simulink model "dec_dly_comp"  (R2023b)
settings: Solver=VariableStepDiscrete  StartTime=0.0  StopTime=DDC_LINEUP_param.endTime  RelTol=1e-3  EnableMultiTasking=on
PreLoadFcn:
  | % Run the setup script when the model is opened
  | setup_dec_dly_comp;
InitFcn:
  | % Run the setup script again just before the
  | % model is run, so that any updates made
  | % after opening are applied.
  | 
  | setup_dec_dly_comp;
StopFcn:
  | dec_dly_comp_output_analysis;
undefined symbols (not defined in the file or in its folder): AdvDSPBChannelOutDisplay, AdvDSPBDMemDisplay, DDC_LINEUP_param, dpoly, dspba_ChannelInVis, dspba_ChannelOutVis, dspba_internal_get_channel_ports, evalAionMaskParam, latency, primtype, UseDontCare, value
libraries: DSPBAPrim x52, DSPBAModelBus x14, DSPBABase x10, simulink x9, DSPBAFilters x2
(part 1 of 2)
Description:
  | DSP Builder Advanced Template for Template Design implementing ModelIP designs
settings Model: Creator=mjervis  LastModifiedBy=5g
settings SolverCC: AlgebraicLoopSolver=TrustRegion
settings DataIOCC: LimitDataPoints=on  SaveFormat=Array  SignalLoggingSaveFormat=ModelDataLogs  ReturnWorkspaceOutputs=off
settings OptimizationCC: ExpressionDepthLimit=2147483647  LifeSpan=inf
settings DebuggingCC: UnderspecifiedInitializationDetection=Classic  MergeDetectMultiDrivingBlocksExec=none  SolverPrmCheckMsg=warning  InheritedTsInSrcMsg=none  IntegerOverflowMsg=none  FcnCallInpInsideContextMsg=warning  UnconnectedInputMsg=warning  UnconnectedOutputMsg=warning  UnconnectedLineMsg=warning  StateNameClashWarn=warning  SFUnexpectedBacktrackingDiag=warning  SFNoUnconditionalDefaultTransitionDiag=warning  SFExecutionAtInitializationDiag=none  IntegerSaturationMsg=none  ArithmeticOperatorsInVariantConditions=warning
settings HardwareCC: ProdBitPerPointer=32  ProdBitPerSizeT=32  ProdBitPerPtrDiffT=32  ProdLargestAtomicFloat=None  ProdIntDivRoundTo=Undefined  ProdEndianess=Unspecified  ProdWordSize=32  ProdHWDeviceType=32-bit Generic
settings ModelReferenceCC: EnableRefExpFcnMdlSchedulingChecks=on  PropagateSignalLabelsOutOfModel=off
settings SFSimCC: SimUseLocalCustomCode=off  CustomCodeUndefinedFunction=UseInterfaceOnly
settings RTWCC: RTWUseLocalCustomCode=off  DLArmComputeVersion=19.05
settings CodeAppCC: StateflowObjectComments=on
settings GRTTargetCC: TargetLangStandard=C89/C90 (ANSI)  CombineOutputUpdateFcns=off  GRTInterface=on
settings ConfigComp: CovMetricSettings=dw  CovSaveCumulativeToWorkspaceVar=on  CovSaveSingleToWorkspaceVar=on  CovExternalEMLEnable=off

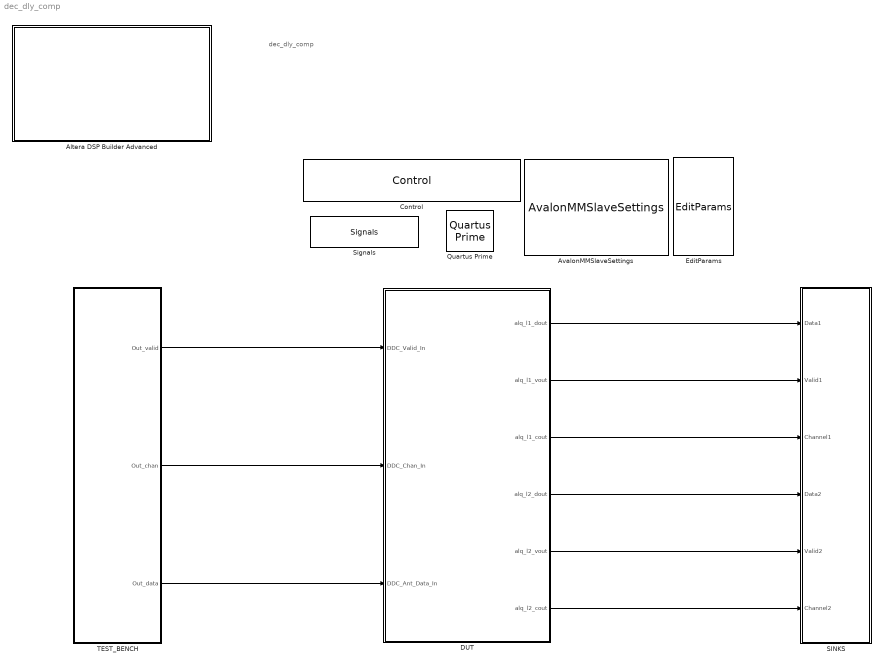
== system dec_dly_comp ==
  note: dec_dly_comp
  Altera DSP Builder Advanced : Subsystem  mask(DSP Builder Advanced Blockset Ignored Block){}
      settings: OpenFcn=web('http://www.altera.com', '-new');
      mask Display: image(imread('intellogo.tif'));
  AvalonMMSlaveSettings : DSPBABase/AvalonMMSlaveSettings
  Control : DSPBABase/Control  generate=on  language=VHDL  destination=./rtl  destination_gui=./rtl  make_full_path=off  path_is_relative=on  autotestbench=on  signaldepth=2  coveragetestbench=off  logs=off  spacewidth=2  spacenum=1  addrwidth=14  datawidth=32  dataendian=Big Endian  hierarchicalnames=off  ramThresholdBits=-1  distRamThresholdBits=-1  mlabThresholdBits=-1  hardMultiplierThresholdLuts=-1  version=20090407  errorOnChanMismatch=1  errorOnGPIOMismatch=0  importModelsimResults=0  cycleAccurate=off  reinterpretCastMult=off  paramFile=dec_dly_comp_params.xml
  DUT : Subsystem
  EditParams : DSPBABase/EditParams  version=20090407
  Quartus Prime : DSPBABase/Quartus Prime  version=20090407
  SINKS : Subsystem
  Signals : DSPBABase/Signals  clk=clk  freq=240  margin=0  rst=areset  rstactive=High  bus=bus  enbusclock=off  busfreq=491.52  bussync=off  version=20090407
  TEST_BENCH : Subsystem
  wires:
  DUT/1(alq_l1_dout) -> SINKS/1(Data1)
  DUT/2(alq_l1_vout) -> SINKS/2(Valid1)
  DUT/3("alq_l1_cout ") -> SINKS/3(Channel1)
  DUT/4(alq_l2_dout) -> SINKS/4(Data2)
  DUT/5(alq_l2_vout) -> SINKS/5(Valid2)
  DUT/6(alq_l2_cout) -> SINKS/6(Channel2)
  TEST_BENCH/1(Out_valid) -> DUT/1(DDC_Valid_In)
  TEST_BENCH/2(Out_chan) -> DUT/2(DDC_Chan_In)
  TEST_BENCH/3(Out_data) -> DUT/3(DDC_Ant_Data_In)

== system dec_dly_comp/Altera DSP Builder Advanced ==

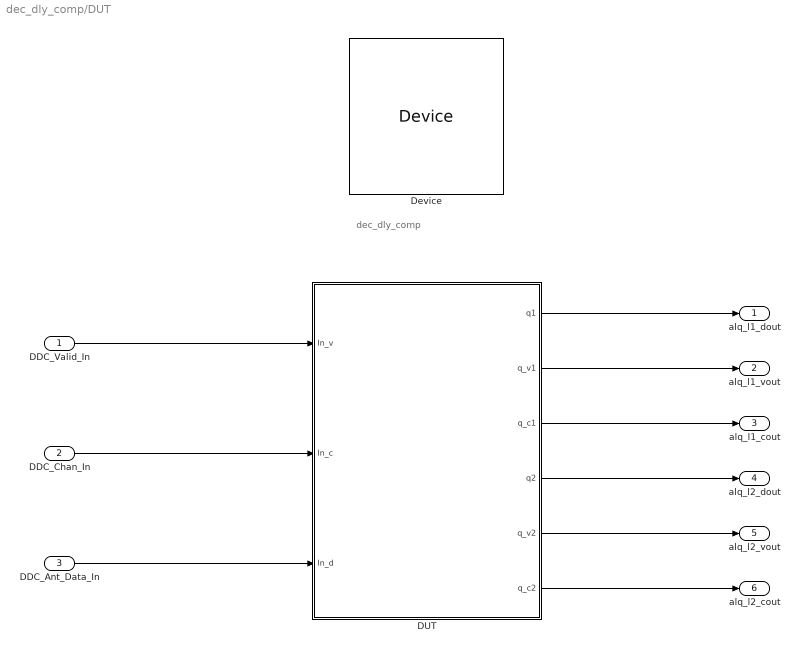
== system dec_dly_comp/DUT ==
  note: dec_dly_comp
  DDC_Valid_In : Inport
  DDC_Chan_In : Inport  Port=2
  DDC_Ant_Data_In : Inport  Port=3
  DUT : Subsystem
  Device : DSPBABase/Device  family=Arria 10  deviceMember=Stratix V GX  stratix4device=Stratix IV GX  hardcopy4device=HardCopy IV E  stratix5device=Stratix V GX  device=10AS066N2F40I1SGES  speed=1  stratixSpeed=-5  stratix2Speed=-3  stratix3Speed=-3  stratix4gxSpeed=-2  stratix4gtSpeed=-1  cyclone2Speed=-6  cyclone3Speed=-7  arria2Speed=-4  cyclone4eSpeed=-8  stratix5Speed=-3  arria5Speed=-4  arriaSpeed=-6  cyclone3lsSpeed=-7  cyclone5Speed=-6  arria2gzSpeed=-3  nightFurySpeed=-2  ecp2Speed=-7  hardcopycompat=off  version=20140217  max10flashmode=off  max10nomeminit=off
  alq_l1_dout : Outport
  alq_l1_vout : Outport  Port=2
  "alq_l1_cout " : Outport  Port=3
  alq_l2_dout : Outport  Port=4
  alq_l2_vout : Outport  Port=5
  alq_l2_cout : Outport  Port=6
  wires:
  DDC_Valid_In/1 -> DUT/1(In_v)
  DDC_Chan_In/1 -> DUT/2(In_c)
  DDC_Ant_Data_In/1 -> DUT/3(In_d)
  DUT/2(q_v1) -> alq_l1_vout/1
  DUT/1(q1) -> alq_l1_dout/1
  DUT/3(q_c1) -> "alq_l1_cout "/1
  DUT/5(q_v2) -> alq_l2_vout/1
  DUT/6(q_c2) -> alq_l2_cout/1
  DUT/4(q2) -> alq_l2_dout/1

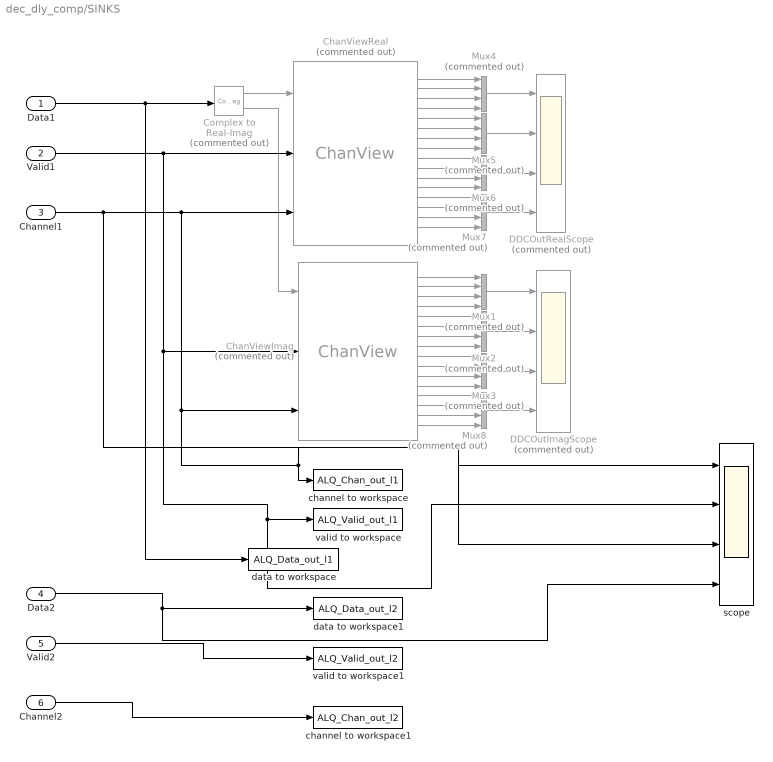
== system dec_dly_comp/SINKS ==
  Data1 : Inport
  Valid1 : Inport  Port=2
  Channel1 : Inport  Port=3
  Data2 : Inport  Port=4
  Valid2 : Inport  Port=5
  Channel2 : Inport  Port=6
  ChanViewImag : DSPBABase/ChanView  Commented=on  nchans=16  chan_vector=[0:15]  outsvalid=off  latency=1  version=20090407
  ChanViewReal : DSPBABase/ChanView  Commented=on  nchans=16  chan_vector=[0:15]  outsvalid=off  latency=1  version=20090407
  Complex to Real-Imag : ComplexToRealImag  Commented=on
  DDCOutImagScope : Scope  Commented=on  NumInputPorts=4
  DDCOutRealScope : Scope  Commented=on  NumInputPorts=4
  Mux{1..8} (8 alike) : Mux  Commented=on
  channel to workspace : ToWorkspace  VariableName=ALQ_Chan_out_l1  SaveFormat=Timeseries  SampleTime=-1
  channel to workspace1 : ToWorkspace  VariableName=ALQ_Chan_out_l2  SaveFormat=Timeseries  SampleTime=-1
  data to workspace : ToWorkspace  VariableName=ALQ_Data_out_l1  SaveFormat=Timeseries  SampleTime=-1
  data to workspace1 : ToWorkspace  VariableName=ALQ_Data_out_l2  SaveFormat=Timeseries  SampleTime=-1
  scope : Scope  NumInputPorts=4
  valid to workspace : ToWorkspace  VariableName=ALQ_Valid_out_l1  SaveFormat=Timeseries  SampleTime=-1
  valid to workspace1 : ToWorkspace  VariableName=ALQ_Valid_out_l2  SaveFormat=Timeseries  SampleTime=-1
  wires:
  Mux7/1 -> DDCOutRealScope/4
  ChanViewReal/14 -> Mux7/2
  ChanViewReal/15 -> Mux7/3
  ChanViewReal/16 -> Mux7/4
  ChanViewReal/13 -> Mux7/1
  Mux6/1 -> DDCOutRealScope/3
  ChanViewReal/11 -> Mux6/3
  ChanViewReal/12 -> Mux6/4
  ChanViewReal/9 -> Mux6/1
  ChanViewReal/10 -> Mux6/2
  Mux5/1 -> DDCOutRealScope/2
  ChanViewReal/6 -> Mux5/2
  ChanViewReal/7 -> Mux5/3
  ChanViewReal/5 -> Mux5/1
  ChanViewReal/8 -> Mux5/4
  Mux4/1 -> DDCOutRealScope/1
  ChanViewReal/3 -> Mux4/3
  ChanViewReal/4 -> Mux4/4
  ChanViewReal/2 -> Mux4/2
  ChanViewReal/1 -> Mux4/1
  Complex to Real-Imag/2 -> ChanViewImag/1
  Complex to Real-Imag/1 -> ChanViewReal/1
  Data1/1 -> data to workspace/1, Complex to Real-Imag/1
  Channel1/1 -> scope/3, scope/1, channel to workspace/1, ChanViewImag/3, ChanViewReal/3
  Valid1/1 -> ChanViewReal/2, scope/2, valid to workspace/1, ChanViewImag/2
  Mux8/1 -> DDCOutImagScope/4
  ChanViewImag/14 -> Mux8/2
  ChanViewImag/15 -> Mux8/3
  ChanViewImag/16 -> Mux8/4
  ChanViewImag/13 -> Mux8/1
  Mux3/1 -> DDCOutImagScope/3
  ChanViewImag/11 -> Mux3/3
  ChanViewImag/12 -> Mux3/4
  ChanViewImag/9 -> Mux3/1
  ChanViewImag/10 -> Mux3/2
  Mux2/1 -> DDCOutImagScope/2
  ChanViewImag/6 -> Mux2/2
  ChanViewImag/7 -> Mux2/3
  ChanViewImag/5 -> Mux2/1
  ChanViewImag/8 -> Mux2/4
  Mux1/1 -> DDCOutImagScope/1
  ChanViewImag/3 -> Mux1/3
  ChanViewImag/4 -> Mux1/4
  ChanViewImag/2 -> Mux1/2
  ChanViewImag/1 -> Mux1/1
  Data2/1 -> scope/4, data to workspace1/1
  Valid2/1 -> valid to workspace1/1
  Channel2/1 -> channel to workspace1/1

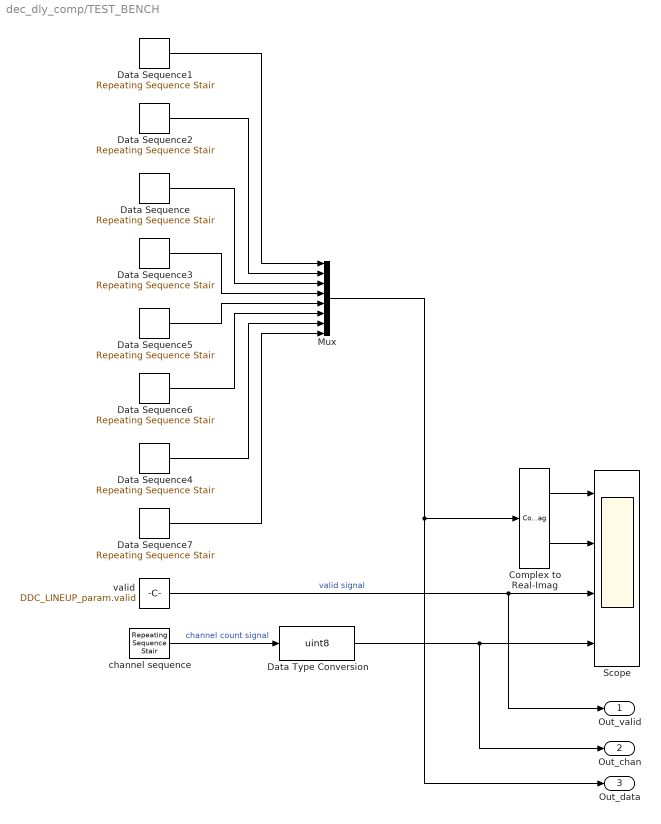
== system dec_dly_comp/TEST_BENCH ==
  Complex to Real-Imag : ComplexToRealImag
  Data Sequence : simulink/Sources/Repeating Sequence Stair  OutValues=DDC_LINEUP_param.DDC_Ant_Data_in_3  tsamp=DDC_LINEUP_param.SampleTime  OutMin=[]  OutMax=[]  OutDataTypeStr=fixdt(1,16,14)  OutputDataTypeScalingMode=Specify via dialog  OutDataType=fixdt(1,16,14)  ConRadixGroup=Best Precision: Vector-wise  OutScaling=[]
  Data Sequence1 : simulink/Sources/Repeating Sequence Stair  OutValues=DDC_LINEUP_param.DDC_Ant_Data_in_1  tsamp=DDC_LINEUP_param.SampleTime  OutMin=[]  OutMax=[]  OutDataTypeStr=fixdt(1,16,14)  OutputDataTypeScalingMode=Specify via dialog  OutDataType=fixdt(1,16,14)  ConRadixGroup=Best Precision: Vector-wise  OutScaling=[]
  Data Sequence2 : simulink/Sources/Repeating Sequence Stair  OutValues=DDC_LINEUP_param.DDC_Ant_Data_in_2  tsamp=DDC_LINEUP_param.SampleTime  OutMin=[]  OutMax=[]  OutDataTypeStr=fixdt(1,16,14)  OutputDataTypeScalingMode=Specify via dialog  OutDataType=fixdt(1,16,14)  ConRadixGroup=Best Precision: Vector-wise  OutScaling=[]
  Data Sequence3 : simulink/Sources/Repeating Sequence Stair  OutValues=DDC_LINEUP_param.DDC_Ant_Data_in_4  tsamp=DDC_LINEUP_param.SampleTime  OutMin=[]  OutMax=[]  OutDataTypeStr=fixdt(1,16,14)  OutputDataTypeScalingMode=Specify via dialog  OutDataType=fixdt(1,16,14)  ConRadixGroup=Best Precision: Vector-wise  OutScaling=[]
  Data Sequence4 : simulink/Sources/Repeating Sequence Stair  OutValues=DDC_LINEUP_param.DDC_Ant_Data_in_7  tsamp=DDC_LINEUP_param.SampleTime  OutMin=[]  OutMax=[]  OutDataTypeStr=fixdt(1,16,14)  OutputDataTypeScalingMode=Specify via dialog  OutDataType=fixdt(1,16,14)  ConRadixGroup=Best Precision: Vector-wise  OutScaling=[]
  Data Sequence5 : simulink/Sources/Repeating Sequence Stair  OutValues=DDC_LINEUP_param.DDC_Ant_Data_in_5  tsamp=DDC_LINEUP_param.SampleTime  OutMin=[]  OutMax=[]  OutDataTypeStr=fixdt(1,16,14)  OutputDataTypeScalingMode=Specify via dialog  OutDataType=fixdt(1,16,14)  ConRadixGroup=Best Precision: Vector-wise  OutScaling=[]
  Data Sequence6 : simulink/Sources/Repeating Sequence Stair  OutValues=DDC_LINEUP_param.DDC_Ant_Data_in_6  tsamp=DDC_LINEUP_param.SampleTime  OutMin=[]  OutMax=[]  OutDataTypeStr=fixdt(1,16,14)  OutputDataTypeScalingMode=Specify via dialog  OutDataType=fixdt(1,16,14)  ConRadixGroup=Best Precision: Vector-wise  OutScaling=[]
  Data Sequence7 : simulink/Sources/Repeating Sequence Stair  OutValues=DDC_LINEUP_param.DDC_Ant_Data_in_8  tsamp=DDC_LINEUP_param.SampleTime  OutMin=[]  OutMax=[]  OutDataTypeStr=fixdt(1,16,14)  OutputDataTypeScalingMode=Specify via dialog  OutDataType=fixdt(1,16,14)  ConRadixGroup=Best Precision: Vector-wise  OutScaling=[]
  Data Type Conversion : DataTypeConversion  OutDataTypeStr=uint8  SaturateOnIntegerOverflow=off  RndMeth=Floor
  Mux : Mux  Inputs=8
  Scope : Scope  NumInputPorts=4
  channel sequence : simulink/Sources/Repeating Sequence Stair  OutValues=DDC_LINEUP_param.channel  tsamp=DDC_LINEUP_param.SampleTime  OutMin=[]  OutMax=[]  OutDataTypeStr=uint8  OutputDataTypeScalingMode=uint8  OutDataType=fixdt(1,16)  ConRadixGroup=Best Precision: Vector-wise  OutScaling=[]
  valid : Constant  Value=DDC_LINEUP_param.valid  OutDataTypeStr=boolean  SampleTime=DDC_LINEUP_param.SampleTime
  Out_valid : Outport
  Out_chan : Outport  Port=2
  Out_data : Outport  Port=3
  wires:
  Complex to Real-Imag/1 -> Scope/1
  valid/1 -> Scope/3, Out_valid/1  "valid signal"
  channel sequence/1 -> Data Type Conversion/1  "channel count signal"
  Data Type Conversion/1 -> Scope/4, Out_chan/1
  Complex to Real-Imag/2 -> Scope/2
  Mux/1 -> Complex to Real-Imag/1, Out_data/1
  Data Sequence5/1 -> Mux/5
  Data Sequence3/1 -> Mux/4
  Data Sequence6/1 -> Mux/6
  Data Sequence/1 -> Mux/3
  Data Sequence4/1 -> Mux/7
  Data Sequence2/1 -> Mux/2
  Data Sequence7/1 -> Mux/8
  Data Sequence1/1 -> Mux/1

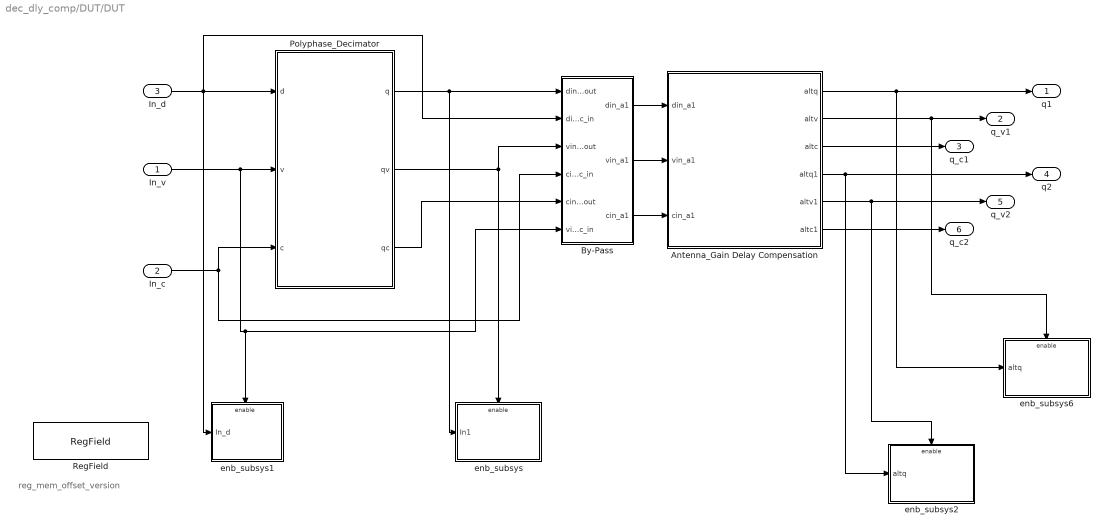
== system dec_dly_comp/DUT/DUT ==
  note: reg_mem_offset_version
  In_v : Inport
  In_c : Inport  Port=2
  In_d : Inport  Port=3
  Antenna_Gain Delay Compensation : Subsystem
  By-Pass : Subsystem
  Polyphase_Decimator : Subsystem
  RegField : DSPBAModelBus/RegField  reg_name=DDC_LINEUP_param.reg_version.mem_offset  reg_rwmode=Read/Write  reg_msb=31  reg_lsb=0  reg_mode=Specify via dialog  reg_type=ufix(32)  reg_scale=2^0  reg_init=DDC_LINEUP_param.reg_version.Version_reg_val  reg_desc=Version_Output  reg_modal=off  reg_desc0=0  reg_desc1=0  reg_desc2=0  reg_desc3=0  reg_desc4=0  reg_desc5=0  reg_desc6=0  reg_desc7=0  reg_addr=13  SampleTime=-1  version=20090407
  enb_subsys : Subsystem
  enb_subsys1 : Subsystem
  enb_subsys2 : Subsystem
  enb_subsys6 : Subsystem
  q1 : Outport
  q_v1 : Outport  Port=2
  q_c1 : Outport  Port=3
  q2 : Outport  Port=4
  q_v2 : Outport  Port=5
  q_c2 : Outport  Port=6
  wires:
  Polyphase_Decimator/2(qv) -> enb_subsys/Enable, By-Pass/3(vin_dec_out)
  Polyphase_Decimator/1(q) -> enb_subsys/1(In1), By-Pass/1(din_dec_out)
  In_d/1 -> By-Pass/2(din_dec_in), enb_subsys1/1(In_d), Polyphase_Decimator/1(d)
  In_v/1 -> enb_subsys1/Enable, By-Pass/6(vin_dec_in), Polyphase_Decimator/2(v)
  In_c/1 -> By-Pass/4(cin_dec_in), Polyphase_Decimator/3(c)
  Antenna_Gain Delay Compensation/3(altc) -> q_c1/1
  Antenna_Gain Delay Compensation/2(altv) -> enb_subsys6/Enable, q_v1/1
  Antenna_Gain Delay Compensation/1(altq) -> enb_subsys6/1(altq), q1/1
  Polyphase_Decimator/3(qc) -> By-Pass/5(cin_dec_out)
  By-Pass/1(din_a1) -> Antenna_Gain Delay Compensation/1(din_a1)
  By-Pass/2(vin_a1) -> Antenna_Gain Delay Compensation/2(vin_a1)
  By-Pass/3(cin_a1) -> Antenna_Gain Delay Compensation/3(cin_a1)
  Antenna_Gain Delay Compensation/4(altq1) -> enb_subsys2/1(altq), q2/1
  Antenna_Gain Delay Compensation/5(altv1) -> enb_subsys2/Enable, q_v2/1
  Antenna_Gain Delay Compensation/6(altc1) -> q_c2/1

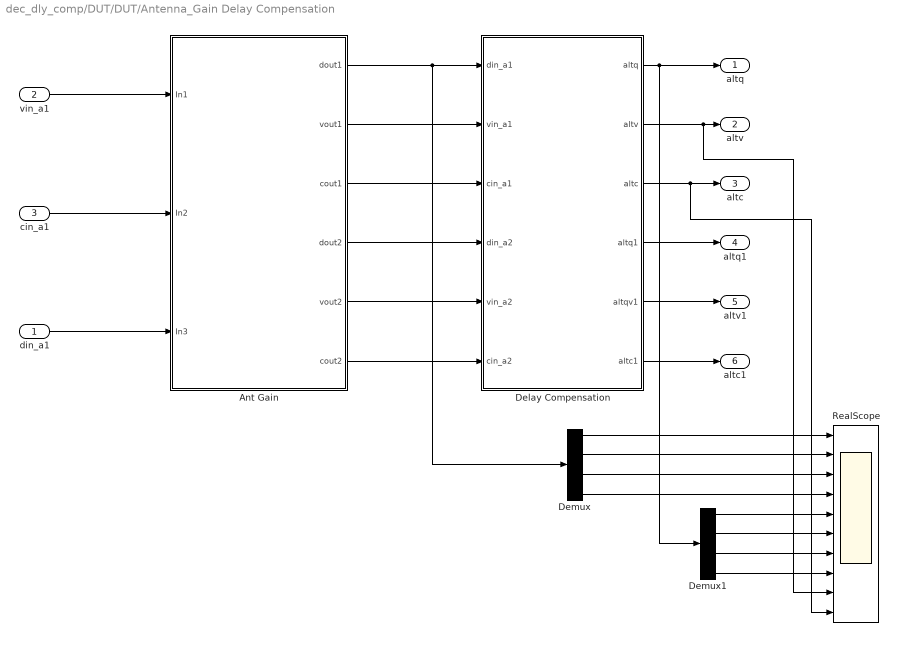
== system dec_dly_comp/DUT/DUT/Antenna_Gain Delay Compensation ==
  din_a1 : Inport
  vin_a1 : Inport  Port=2
  cin_a1 : Inport  Port=3
  Ant Gain : Subsystem
  Delay Compensation : Subsystem
  Demux : Demux
  Demux1 : Demux
  RealScope : Scope  NumInputPorts=10
  altq : Outport
  altv : Outport  Port=2
  altc : Outport  Port=3
  altq1 : Outport  Port=4
  altv1 : Outport  Port=5
  altc1 : Outport  Port=6
  wires:
  vin_a1/1 -> Ant Gain/1(In1)
  cin_a1/1 -> Ant Gain/2(In2)
  din_a1/1 -> Ant Gain/3(In3)
  Ant Gain/3(cout1) -> Delay Compensation/3(cin_a1)
  Ant Gain/2(vout1) -> Delay Compensation/2(vin_a1)
  Ant Gain/4(dout2) -> Delay Compensation/4(din_a2)
  Ant Gain/5(vout2) -> Delay Compensation/5(vin_a2)
  Ant Gain/6(cout2) -> Delay Compensation/6(cin_a2)
  Delay Compensation/4(altq1) -> altq1/1
  Delay Compensation/5(altqv1) -> altv1/1
  Delay Compensation/6(altc1) -> altc1/1
  Ant Gain/1(dout1) -> Demux/1, Delay Compensation/1(din_a1)
  Demux1/2 -> RealScope/6
  Demux/2 -> RealScope/2
  Delay Compensation/2(altv) -> RealScope/9, altv/1
  Demux/1 -> RealScope/1
  Demux1/1 -> RealScope/5
  Demux1/4 -> RealScope/8
  Demux/4 -> RealScope/4
  Demux/3 -> RealScope/3
  Delay Compensation/3(altc) -> RealScope/10, altc/1
  Demux1/3 -> RealScope/7
  Delay Compensation/1(altq) -> altq/1, Demux1/1

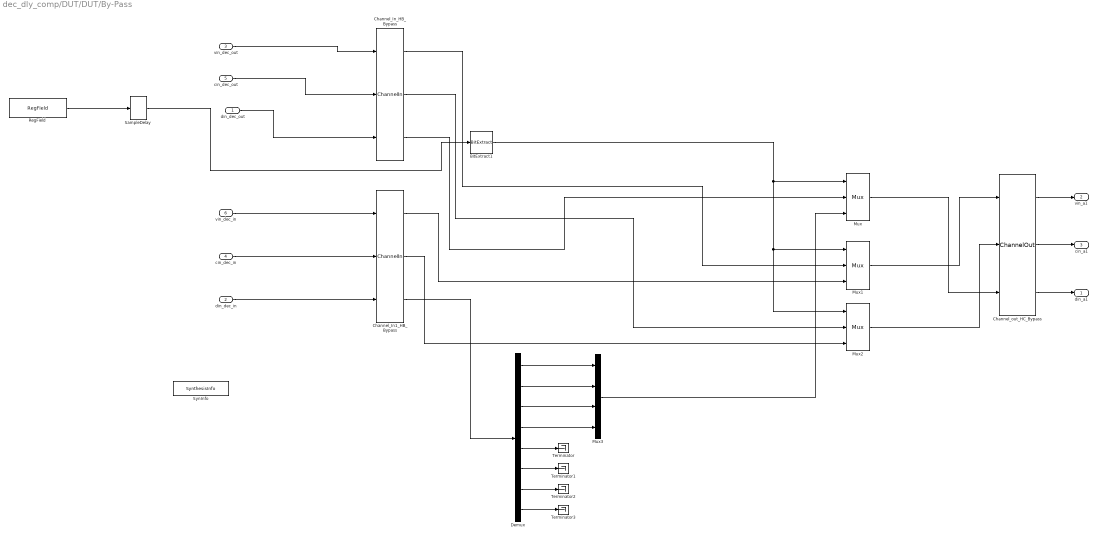
== system dec_dly_comp/DUT/DUT/By-Pass ==
  din_dec_out : Inport
  din_dec_in : Inport  Port=2
  vin_dec_out : Inport  Port=3
  cin_dec_in : Inport  Port=4
  cin_dec_out : Inport  Port=5
  vin_dec_in : Inport  Port=6
  BitExtract1 : DSPBAPrim/BitExtract  primtype=bitextract  nInputs=1  nOutputs=1  omode=boolean  otype=uint(16)  scale=1  rndmethod=Unbiased  factor=1  satmethod=Symmetric  shift_vec=[0 1 2 -1]  value=0  inPortNames=[' '; ' ';]  outPortNames=[' ']  dspbaimage=dspba_prim.svg  text=fprintf('..%d', value);  style=Optimised  visibilities=8+1024  version=20211007
  Channel_In1_HB_Bypass : DSPBAPrim/ChannelIn  primtype=channelin  nInputs=dspba_internal_get_channel_ports(gcb)  nOutputs=dspba_internal_get_channel_ports(gcb)  omode=Inherit via internal rule  otype=sfix(16)  scale=2^-15  rndmethod=Unbiased  factor=1  satmethod=Symmetric  shift_vec=[0 1 2 -1]  value=1  inPortNames=['v'; 'c'; '0'; '1'; '2'; '3'; '4'; '5'; '6'; '7'; '8'; '9'; 'A'; 'B'; 'D'; 'E'; 'F'; 'G'; 'H'; 'I'; 'J'; 'K'; 'L'; 'M'; 'N'; 'O'; 'P'; 'Q'; 'R'; 'S'; 'T'; 'U'; 'W'; 'X'; 'Y'; 'Z']  outPortNames=['v'; 'c'; '0'; '1'; '2'; '3'; '4'; '5'; '6'; '7'; '8'; '9'; 'A'; 'B'; 'D'; 'E'; 'F'; 'G'; 'H'; 'I'; 'J'; 'K'; 'L'; 'M'; 'N'; 'O'; 'P'; 'Q'; 'R'; 'S'; 'T'; 'U'; 'W'; 'X'; 'Y'; 'Z']  dspbaimage=dspba_prim_channel_tall.svg  text=fprintf('In');  style=Optimised  dataSignals=1  foldingEnabled=off  channels=1  sampleRate=200  packetBeginPresent=off  packetBeginEnabled=off  visibilities=dspba_ChannelInVis(gcb)  scheduleOrigin=on  version=20211214
  Channel_In_HB_Bypass : DSPBAPrim/ChannelIn  primtype=channelin  nInputs=dspba_internal_get_channel_ports(gcb)  nOutputs=dspba_internal_get_channel_ports(gcb)  omode=Inherit via internal rule  otype=sfix(16)  scale=2^-15  rndmethod=Unbiased  factor=1  satmethod=Symmetric  shift_vec=[0 1 2 -1]  value=1  inPortNames=['v'; 'c'; '0'; '1'; '2'; '3'; '4'; '5'; '6'; '7'; '8'; '9'; 'A'; 'B'; 'D'; 'E'; 'F'; 'G'; 'H'; 'I'; 'J'; 'K'; 'L'; 'M'; 'N'; 'O'; 'P'; 'Q'; 'R'; 'S'; 'T'; 'U'; 'W'; 'X'; 'Y'; 'Z']  outPortNames=['v'; 'c'; '0'; '1'; '2'; '3'; '4'; '5'; '6'; '7'; '8'; '9'; 'A'; 'B'; 'D'; 'E'; 'F'; 'G'; 'H'; 'I'; 'J'; 'K'; 'L'; 'M'; 'N'; 'O'; 'P'; 'Q'; 'R'; 'S'; 'T'; 'U'; 'W'; 'X'; 'Y'; 'Z']  dspbaimage=dspba_prim_channel_tall.svg  text=fprintf('In');  style=Optimised  dataSignals=1  foldingEnabled=off  channels=1  sampleRate=200  packetBeginPresent=off  packetBeginEnabled=off  visibilities=dspba_ChannelInVis(gcb)  scheduleOrigin=on  version=20211214
  Channel_out_HC_Bypass : DSPBAPrim/ChannelOut  primtype=channelout  nInputs=dspba_internal_get_channel_ports(gcb)  nOutputs=dspba_internal_get_channel_ports(gcb)  omode=Inherit via internal rule  otype=sfix(16)  scale=2^-15  rndmethod=Unbiased  factor=1  satmethod=Symmetric  shift_vec=[0 1 2 -1]  value=1  inPortNames=['v'; 'c'; '0'; '1'; '2'; '3'; '4'; '5'; '6'; '7'; '8'; '9'; 'A'; 'B'; 'D'; 'E'; 'F'; 'G'; 'H'; 'I'; 'J'; 'K'; 'L'; 'M'; 'N'; 'O'; 'P'; 'Q'; 'R'; 'S'; 'T'; 'U'; 'W'; 'X'; 'Y'; 'Z']  outPortNames=['v'; 'c'; '0'; '1'; '2'; '3'; '4'; '5'; '6'; '7'; '8'; '9'; 'A'; 'B'; 'D'; 'E'; 'F'; 'G'; 'H'; 'I'; 'J'; 'K'; 'L'; 'M'; 'N'; 'O'; 'P'; 'Q'; 'R'; 'S'; 'T'; 'U'; 'W'; 'X'; 'Y'; 'Z']  dspbaimage=dspba_prim_channel_tall.svg  text=fprintf('Out%s', AdvDSPBChannelOutDisplay(latency));  style=Optimised  dataSignals=1  foldingEnabled=off  channels=1  sampleRate=200  packetBeginPresent=off  packetBeginEnabled=off  visibilities=dspba_ChannelOutVis(gcb)  latency=0  version=20211214
  Demux : Demux  Outputs=8
  Mux : DSPBAPrim/Mux  primtype=mux  nInputs=evalAionMaskParam(gcb,'value',1)+1  nOutputs=1  omode=Inherit via internal rule  otype=sfix(16)  scale=2^-15  rndmethod=Unbiased  factor=1  satmethod=Symmetric  shift_vec=[0 1 2 -1]  value=2  inPortNames=['s '; 'd0'; 'd1'; 'd2'; 'd3'; 'd4'; 'd5'; 'd6'; 'd7'; 'd8'; 'd9';]  outPortNames=[' ']  dspbaimage=dspba_prim_tall.svg  text=fprintf('%s', primtype);  style=Optimised  visibilities=1032  version=20211007
  Mux1 : DSPBAPrim/Mux  primtype=mux  nInputs=evalAionMaskParam(gcb,'value',1)+1  nOutputs=1  omode=Inherit via internal rule  otype=sfix(16)  scale=2^-15  rndmethod=Unbiased  factor=1  satmethod=Symmetric  shift_vec=[0 1 2 -1]  value=2  inPortNames=['s '; 'd0'; 'd1'; 'd2'; 'd3'; 'd4'; 'd5'; 'd6'; 'd7'; 'd8'; 'd9';]  outPortNames=[' ']  dspbaimage=dspba_prim_tall.svg  text=fprintf('%s', primtype);  style=Optimised  visibilities=1032  version=20211007
  Mux2 : DSPBAPrim/Mux  primtype=mux  nInputs=evalAionMaskParam(gcb,'value',1)+1  nOutputs=1  omode=Inherit via internal rule  otype=sfix(16)  scale=2^-15  rndmethod=Unbiased  factor=1  satmethod=Symmetric  shift_vec=[0 1 2 -1]  value=2  inPortNames=['s '; 'd0'; 'd1'; 'd2'; 'd3'; 'd4'; 'd5'; 'd6'; 'd7'; 'd8'; 'd9';]  outPortNames=[' ']  dspbaimage=dspba_prim_tall.svg  text=fprintf('%s', primtype);  style=Optimised  visibilities=1032  version=20211007
  Mux3 : Mux
  RegField : DSPBAModelBus/RegField  reg_name=DDC_LINEUP_param.HB_Bypass  reg_rwmode=Read/Write  reg_msb=15  reg_lsb=0  reg_mode=Specify via dialog  reg_type=ufix(16)  reg_scale=2^-0  reg_init=0  reg_desc=Description of what is stored in this field  reg_modal=off  reg_desc0=0  reg_desc1=0  reg_desc2=0  reg_desc3=0  reg_desc4=0  reg_desc5=0  reg_desc6=0  reg_desc7=0  reg_addr=4  SampleTime=-1  version=20090407
  SampleDelay : DSPBAPrim/SampleDelay  primtype=sampdelay  nInputs=1  nOutputs=1  omode=Inherit via internal rule  otype=sfix(16)  scale=2^-15  rndmethod=Unbiased  factor=1  satmethod=Symmetric  shift_vec=[0 1 2 -1]  floatPrecision=float32_m23  value=1  inPortNames=[' '; ' ';]  outPortNames=[' ']  dspbaimage=dspba_prim.svg  text=dpoly(1, eye(1,value+1), 'z')  style=Optimised  visibilities=8 + 1024 + 2^17 + 2^18  flexible=off  slackgroup=0  augmented=0  version=20211007  advOptions=[]
  SynInfo : DSPBAPrim/SynthesisInfo  primtype=synthinfo  nInputs=0  nOutputs=0  omode=Inherit via internal rule  otype=sfix(16)  scale=2^-15  rndmethod=Truncate  factor=1  satmethod=Symmetric  shift_vec=[0 1 2 -1]  value=99  inPortNames=[' '; ' ';]  outPortNames=[' ']  dspbaimage=dspba_prim_ctrl.jpg  text=fprintf('Style=%s', style);  style=Scheduled  visibilities=2^17+2^18+2^19+2^20  constraintPair=None  constraintRelation=>  constraintLimit=4  modelRefSign=+  modelRef=''  showSchedule=off  simulationMode=Use Global Value  resetMinimization=Off  version=20220106
  Terminator{,1..3} (4 alike) : Terminator
  din_a1 : Outport
  vin_a1 : Outport  Port=2
  cin_a1 : Outport  Port=3
  wires:
  Channel_out_HC_Bypass/2 -> cin_a1/1
  Channel_out_HC_Bypass/1 -> vin_a1/1
  Channel_out_HC_Bypass/3 -> din_a1/1
  Channel_In1_HB_Bypass/2 -> Mux2/3
  Channel_In_HB_Bypass/3 -> Mux/2
  Channel_In_HB_Bypass/1 -> Mux1/2
  Channel_In_HB_Bypass/2 -> Mux2/2
  Channel_In1_HB_Bypass/1 -> Mux1/3
  Channel_In1_HB_Bypass/3 -> Demux/1
  SampleDelay/1 -> BitExtract1/1
  din_dec_out/1 -> Channel_In_HB_Bypass/3
  din_dec_in/1 -> Channel_In1_HB_Bypass/3
  vin_dec_out/1 -> Channel_In_HB_Bypass/1
  cin_dec_in/1 -> Channel_In1_HB_Bypass/2
  cin_dec_out/1 -> Channel_In_HB_Bypass/2
  vin_dec_in/1 -> Channel_In1_HB_Bypass/1
  Mux/1 -> Channel_out_HC_Bypass/3
  Mux1/1 -> Channel_out_HC_Bypass/1
  Mux2/1 -> Channel_out_HC_Bypass/2
  Mux3/1 -> Mux/3
  BitExtract1/1 -> Mux2/1, Mux1/1, Mux/1
  Demux/1 -> Mux3/1
  Demux/2 -> Mux3/2
  Demux/3 -> Mux3/3
  Demux/4 -> Mux3/4
  Demux/5 -> Terminator/1
  Demux/6 -> Terminator1/1
  Demux/8 -> Terminator3/1
  Demux/7 -> Terminator2/1
  RegField/1 -> SampleDelay/1

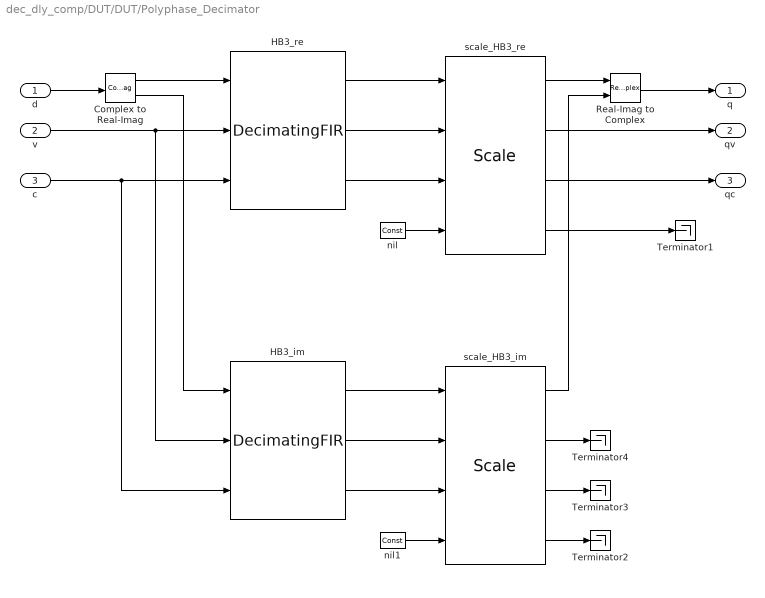
== system dec_dly_comp/DUT/DUT/Polyphase_Decimator ==
  d : Inport
  v : Inport  Port=2
  c : Inport  Port=3
  Complex to Real-Imag : ComplexToRealImag
  HB3_im : DSPBAFilters/DecimatingFIR  nInputRate=DDC_LINEUP_param.HB_filter3.SampleRate  decim=DDC_LINEUP_param.HB_filter3.Decimation  nchan=DDC_LINEUP_param.HB_filter3.ChanCount  symmetry=Symmetrical  coef=DDC_LINEUP_param.HB_filt3.coeffs  addr=DDC_LINEUP_param.HB_filter6_3.base_addr  rwmode=Constant  nband=Half Band  exposebus=off  latency=25  version=20090407  recon=off  MM=[0,1,2,3,4,5,6,7,8,9,10,11,12,13,14,15]  resetrezero=off  sharecoef=auto  simulationMode=Standard
  HB3_re : DSPBAFilters/DecimatingFIR  nInputRate=DDC_LINEUP_param.HB_filter3.SampleRate  decim=DDC_LINEUP_param.HB_filter3.Decimation  nchan=DDC_LINEUP_param.HB_filter3.ChanCount  symmetry=Symmetrical  coef=DDC_LINEUP_param.HB_filt3.coeffs  addr=DDC_LINEUP_param.HB_filter6_3.base_addr  rwmode=Constant  nband=Half Band  exposebus=off  latency=25  version=20090407  recon=off  MM=[0,1,2,3,4,5,6,7,8,9,10,11,12,13,14,15]  resetrezero=off  sharecoef=auto  simulationMode=Standard
  Real-Imag to Complex : RealImagToComplex
  Terminator{1..4} (4 alike) : Terminator
  nil : DSPBAPrim/Const  primtype=const  nInputs=0  nOutputs=1  omode=Inherit via internal rule  otype=sfix(16)  scale=2^-15  rndmethod=Unbiased  factor=1  satmethod=Symmetric  shift_vec=[0 1 2 -1]  value=0  inPortNames=['+'; '+';]  outPortNames=[' ']  dspbaimage=dspba_prim.svg  text=fprintf('%s', num2str(value));  style=Optimised  visibilities=8 + 1024  floatPrecision=float32_m23  warnSaturation=on  version=20211007  SampleTime=inf
  nil1 : DSPBAPrim/Const  primtype=const  nInputs=0  nOutputs=1  omode=Inherit via internal rule  otype=sfix(16)  scale=2^-15  rndmethod=Unbiased  factor=1  satmethod=Symmetric  shift_vec=[0 1 2 -1]  value=0  inPortNames=['+'; '+';]  outPortNames=[' ']  dspbaimage=dspba_prim.svg  text=fprintf('%s', num2str(value));  style=Optimised  visibilities=8 + 1024  floatPrecision=float32_m23  warnSaturation=on  version=20211007  SampleTime=inf
  scale_HB3_im : DSPBABase/Scale  otype=sfix(DDC_LINEUP_param.output_word_length)  scale=2^-DDC_LINEUP_param.output_fraction_length  rndmethod=Biased  factor=1  satmethod=None  shift_vec=0  latency=2  simulationMode=Use Global Value  version=20130807
  scale_HB3_re : DSPBABase/Scale  otype=sfix(DDC_LINEUP_param.output_word_length)  scale=2^-DDC_LINEUP_param.output_fraction_length  rndmethod=Biased  factor=1  satmethod=None  shift_vec=0  latency=2  simulationMode=Use Global Value  version=20130807
  q : Outport
  qv : Outport  Port=2
  qc : Outport  Port=3
  wires:
  scale_HB3_re/1 -> Real-Imag to Complex/1
  HB3_re/3 -> scale_HB3_re/3
  c/1 -> HB3_im/3, HB3_re/3
  scale_HB3_re/3 -> qc/1
  scale_HB3_re/2 -> qv/1
  HB3_re/2 -> scale_HB3_re/2
  v/1 -> HB3_im/2, HB3_re/2
  nil1/1 -> scale_HB3_im/4
  scale_HB3_re/4 -> Terminator1/1
  HB3_re/1 -> scale_HB3_re/1
  Complex to Real-Imag/1 -> HB3_re/1
  nil/1 -> scale_HB3_re/4
  d/1 -> Complex to Real-Imag/1
  scale_HB3_im/4 -> Terminator2/1
  HB3_im/1 -> scale_HB3_im/1
  scale_HB3_im/1 -> Real-Imag to Complex/2
  scale_HB3_im/2 -> Terminator4/1
  Complex to Real-Imag/2 -> HB3_im/1
  HB3_im/2 -> scale_HB3_im/2
  scale_HB3_im/3 -> Terminator3/1
  Real-Imag to Complex/1 -> q/1
  HB3_im/3 -> scale_HB3_im/3

== system dec_dly_comp/DUT/DUT/enb_subsys ==
  In1 : Inport
  Enable : EnablePort
  To Workspace : ToWorkspace  VariableName=polyphase_dec_dout  SampleTime=-1
      settings: Save2DSignal=2-D array (concatenate along first dimension)
  wires:
  In1/1 -> To Workspace/1

== system dec_dly_comp/DUT/DUT/enb_subsys1 ==
  In_d : Inport
  Enable : EnablePort
  To Workspace : ToWorkspace  VariableName=polyphase_dec_din  SampleTime=-1
      settings: Save2DSignal=2-D array (concatenate along first dimension)
  wires:
  In_d/1 -> To Workspace/1

== system dec_dly_comp/DUT/DUT/enb_subsys2 ==
  altq : Inport
  Enable : EnablePort
  To Workspace : ToWorkspace  VariableName=decimator_out_dspba2  SampleTime=-1
      settings: Save2DSignal=2-D array (concatenate along first dimension)
  wires:
  altq/1 -> To Workspace/1

== system dec_dly_comp/DUT/DUT/enb_subsys6 ==
  altq : Inport
  Enable : EnablePort
  To Workspace : ToWorkspace  VariableName=decimator_out_dspba1  SampleTime=-1
      settings: Save2DSignal=2-D array (concatenate along first dimension)
  wires:
  altq/1 -> To Workspace/1

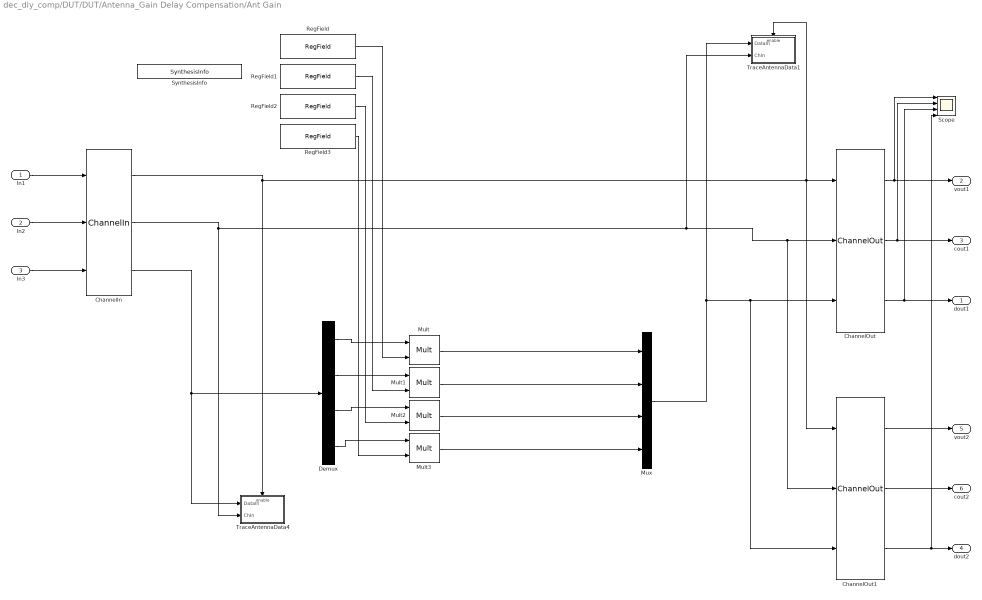
== system dec_dly_comp/DUT/DUT/Antenna_Gain Delay Compensation/Ant Gain ==
  In1 : Inport
  In2 : Inport  Port=2
  In3 : Inport  Port=3
  ChannelIn : DSPBAPrim/ChannelIn  primtype=channelin  nInputs=dspba_internal_get_channel_ports(gcb)  nOutputs=dspba_internal_get_channel_ports(gcb)  omode=Inherit via internal rule  otype=sfix(16)  scale=2^-15  rndmethod=Unbiased  factor=1  satmethod=Symmetric  shift_vec=[0 1 2 -1]  value=1  inPortNames=['v'; 'c'; '0'; '1'; '2'; '3'; '4'; '5'; '6'; '7'; '8'; '9'; 'A'; 'B'; 'D'; 'E'; 'F'; 'G'; 'H'; 'I'; 'J'; 'K'; 'L'; 'M'; 'N'; 'O'; 'P'; 'Q'; 'R'; 'S'; 'T'; 'U'; 'W'; 'X'; 'Y'; 'Z']  outPortNames=['v'; 'c'; '0'; '1'; '2'; '3'; '4'; '5'; '6'; '7'; '8'; '9'; 'A'; 'B'; 'D'; 'E'; 'F'; 'G'; 'H'; 'I'; 'J'; 'K'; 'L'; 'M'; 'N'; 'O'; 'P'; 'Q'; 'R'; 'S'; 'T'; 'U'; 'W'; 'X'; 'Y'; 'Z']  dspbaimage=dspba_prim_channel_tall.svg  text=fprintf('In');  style=Optimised  dataSignals=1  foldingEnabled=off  channels=1  sampleRate=200  packetBeginPresent=off  packetBeginEnabled=off  visibilities=dspba_ChannelInVis(gcb)  scheduleOrigin=on  version=20211214
  ChannelOut : DSPBAPrim/ChannelOut  primtype=channelout  nInputs=dspba_internal_get_channel_ports(gcb)  nOutputs=dspba_internal_get_channel_ports(gcb)  omode=Inherit via internal rule  otype=sfix(16)  scale=2^-15  rndmethod=Unbiased  factor=1  satmethod=Symmetric  shift_vec=[0 1 2 -1]  value=1  inPortNames=['v'; 'c'; '0'; '1'; '2'; '3'; '4'; '5'; '6'; '7'; '8'; '9'; 'A'; 'B'; 'D'; 'E'; 'F'; 'G'; 'H'; 'I'; 'J'; 'K'; 'L'; 'M'; 'N'; 'O'; 'P'; 'Q'; 'R'; 'S'; 'T'; 'U'; 'W'; 'X'; 'Y'; 'Z']  outPortNames=['v'; 'c'; '0'; '1'; '2'; '3'; '4'; '5'; '6'; '7'; '8'; '9'; 'A'; 'B'; 'D'; 'E'; 'F'; 'G'; 'H'; 'I'; 'J'; 'K'; 'L'; 'M'; 'N'; 'O'; 'P'; 'Q'; 'R'; 'S'; 'T'; 'U'; 'W'; 'X'; 'Y'; 'Z']  dspbaimage=dspba_prim_channel_tall.svg  text=fprintf('Out%s', AdvDSPBChannelOutDisplay(latency));  style=Optimised  dataSignals=1  foldingEnabled=off  channels=1  sampleRate=200  packetBeginPresent=off  packetBeginEnabled=off  visibilities=dspba_ChannelOutVis(gcb)  latency=6  version=20211214
  ChannelOut1 : DSPBAPrim/ChannelOut  primtype=channelout  nInputs=dspba_internal_get_channel_ports(gcb)  nOutputs=dspba_internal_get_channel_ports(gcb)  omode=Inherit via internal rule  otype=sfix(16)  scale=2^-15  rndmethod=Unbiased  factor=1  satmethod=Symmetric  shift_vec=[0 1 2 -1]  value=1  inPortNames=['v'; 'c'; '0'; '1'; '2'; '3'; '4'; '5'; '6'; '7'; '8'; '9'; 'A'; 'B'; 'D'; 'E'; 'F'; 'G'; 'H'; 'I'; 'J'; 'K'; 'L'; 'M'; 'N'; 'O'; 'P'; 'Q'; 'R'; 'S'; 'T'; 'U'; 'W'; 'X'; 'Y'; 'Z']  outPortNames=['v'; 'c'; '0'; '1'; '2'; '3'; '4'; '5'; '6'; '7'; '8'; '9'; 'A'; 'B'; 'D'; 'E'; 'F'; 'G'; 'H'; 'I'; 'J'; 'K'; 'L'; 'M'; 'N'; 'O'; 'P'; 'Q'; 'R'; 'S'; 'T'; 'U'; 'W'; 'X'; 'Y'; 'Z']  dspbaimage=dspba_prim_channel_tall.svg  text=fprintf('Out%s', AdvDSPBChannelOutDisplay(latency));  style=Optimised  dataSignals=1  foldingEnabled=off  channels=1  sampleRate=200  packetBeginPresent=off  packetBeginEnabled=off  visibilities=dspba_ChannelOutVis(gcb)  latency=6  version=20211214
  Demux : Demux
  Mult{,1..3} (4 alike) : DSPBAPrim/Mult  primtype=mult  nInputs=2  nOutputs=1  omode=Inherit via internal rule  otype=sfix(16)  scale=2^-15  rndmethod=Unbiased  factor=1  satmethod=Symmetric  shift_vec=[0 1 2 -1]  value=0  inPortNames=[' '; ' ';]  outPortNames=[' ']  dspbaimage=dspba_prim.svg  text=fprintf('X');  style=Optimised  visibilities=8+2^18+2^19  floatPrecision=float32_m23  floatRounding=correct  advOptions=[]  version=20211007
  Mux : Mux
  RegField : DSPBAModelBus/RegField  reg_name=DDC_Gain_Ant1_offset  reg_rwmode=Read/Write  reg_msb=15  reg_lsb=0  reg_mode=Specify via dialog  reg_type=ufix(16)  reg_scale=2^-13  reg_init=DDC_Gain_Ant1  reg_desc=Digital Gain per Antenna  reg_modal=off  reg_desc0=0  reg_desc1=0  reg_desc2=0  reg_desc3=0  reg_desc4=0  reg_desc5=0  reg_desc6=0  reg_desc7=0  reg_addr=0  SampleTime=-1  version=20090407
  RegField1 : DSPBAModelBus/RegField  reg_name=DDC_Gain_Ant2_offset  reg_rwmode=Read/Write  reg_msb=15  reg_lsb=0  reg_mode=Specify via dialog  reg_type=ufix(16)  reg_scale=2^-13  reg_init=DDC_Gain_Ant2  reg_desc=Digital Gain per Antenna  reg_modal=off  reg_desc0=0  reg_desc1=0  reg_desc2=0  reg_desc3=0  reg_desc4=0  reg_desc5=0  reg_desc6=0  reg_desc7=0  reg_addr=1  SampleTime=-1  version=20090407
  RegField2 : DSPBAModelBus/RegField  reg_name=DDC_Gain_Ant3_offset  reg_rwmode=Read/Write  reg_msb=15  reg_lsb=0  reg_mode=Specify via dialog  reg_type=ufix(16)  reg_scale=2^-13  reg_init=DDC_Gain_Ant3  reg_desc=Digital Gain per Antenna  reg_modal=off  reg_desc0=0  reg_desc1=0  reg_desc2=0  reg_desc3=0  reg_desc4=0  reg_desc5=0  reg_desc6=0  reg_desc7=0  reg_addr=2  SampleTime=-1  version=20090407
  RegField3 : DSPBAModelBus/RegField  reg_name=DDC_Gain_Ant4_offset  reg_rwmode=Read/Write  reg_msb=15  reg_lsb=0  reg_mode=Specify via dialog  reg_type=ufix(16)  reg_scale=2^-13  reg_init=DDC_Gain_Ant4  reg_desc=Digital Gain per Antenna  reg_modal=off  reg_desc0=0  reg_desc1=0  reg_desc2=0  reg_desc3=0  reg_desc4=0  reg_desc5=0  reg_desc6=0  reg_desc7=0  reg_addr=3  SampleTime=-1  version=20090407
  Scope : Scope  NumInputPorts=4
  SynthesisInfo : DSPBAPrim/SynthesisInfo  primtype=synthinfo  nInputs=0  nOutputs=0  omode=Inherit via internal rule  otype=sfix(16)  scale=2^-15  rndmethod=Truncate  factor=1  satmethod=Symmetric  shift_vec=[0 1 2 -1]  value=99  inPortNames=[' '; ' ';]  outPortNames=[' ']  dspbaimage=dspba_prim_ctrl.jpg  text=fprintf('Style=%s', style);  style=Scheduled  visibilities=2^15+2^17+2^18+2^19  constraintPair=None  constraintRelation=>  constraintLimit=Latency  modelRefSign=+  modelRef=''  showSchedule=off  simulationMode=Use Global Value  resetMinimization=Conditional - On for ChannelIn/Out only  version=20220106
  TraceAntennaData1 : Subsystem  TreatAsAtomicUnit=on
  TraceAntennaData4 : Subsystem  TreatAsAtomicUnit=on
  dout1 : Outport
  vout1 : Outport  Port=2
  cout1 : Outport  Port=3
  dout2 : Outport  Port=4
  vout2 : Outport  Port=5
  cout2 : Outport  Port=6
  wires:
  ChannelIn/2 -> TraceAntennaData1/2(ChIn), ChannelOut1/2, ChannelOut/2, TraceAntennaData4/2(ChIn)
  ChannelIn/1 -> TraceAntennaData4/Enable, ChannelOut1/1, ChannelOut/1, TraceAntennaData1/Enable
  ChannelIn/3 -> TraceAntennaData4/1(DataIn), Demux/1
  Mux/1 -> ChannelOut1/3, ChannelOut/3, TraceAntennaData1/1(DataIn)
  Demux/1 -> Mult/1
  Mult/1 -> Mux/1
  Mult3/1 -> Mux/4
  In2/1 -> ChannelIn/2
  ChannelOut/2 -> cout1/1, Scope/2
  In3/1 -> ChannelIn/3
  ChannelOut1/2 -> cout2/1
  ChannelOut/3 -> dout1/1, Scope/3
  RegField1/1 -> Mult1/2
  Demux/3 -> Mult2/1
  Demux/2 -> Mult1/1
  RegField/1 -> Mult/2
  Demux/4 -> Mult3/1
  RegField2/1 -> Mult2/2
  RegField3/1 -> Mult3/2
  Mult1/1 -> Mux/2
  Mult2/1 -> Mux/3
  ChannelOut/1 -> vout1/1, Scope/1
  In1/1 -> ChannelIn/1
  ChannelOut1/1 -> vout2/1
  ChannelOut1/3 -> Scope/4, dout2/1

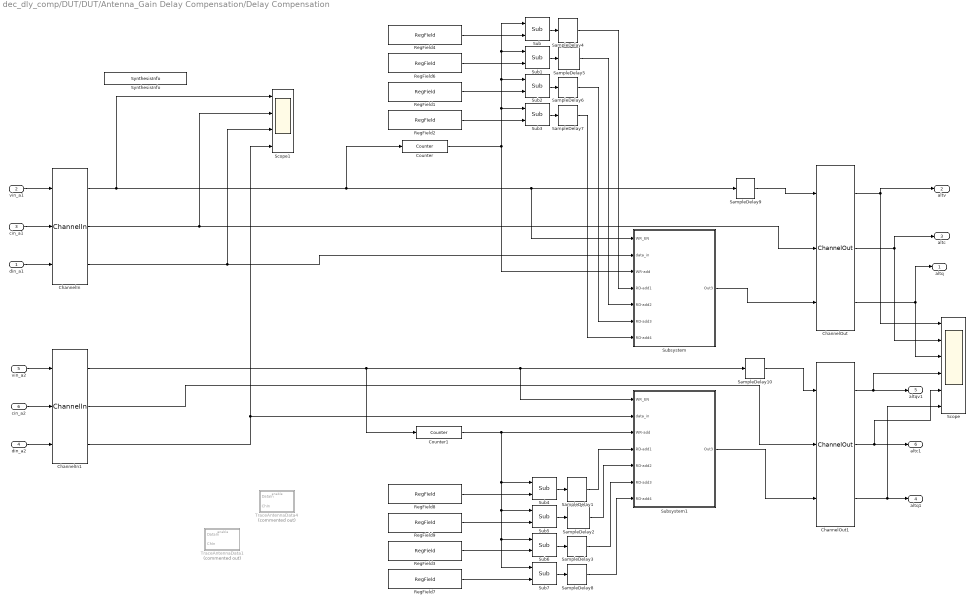
== system dec_dly_comp/DUT/DUT/Antenna_Gain Delay Compensation/Delay Compensation ==
  din_a1 : Inport
  vin_a1 : Inport  Port=2
  cin_a1 : Inport  Port=3
  din_a2 : Inport  Port=4
  vin_a2 : Inport  Port=5
  cin_a2 : Inport  Port=6
  ChannelIn : DSPBAPrim/ChannelIn  primtype=channelin  nInputs=dspba_internal_get_channel_ports(gcb)  nOutputs=dspba_internal_get_channel_ports(gcb)  omode=Inherit via internal rule  otype=sfix(16)  scale=2^-15  rndmethod=Unbiased  factor=1  satmethod=Symmetric  shift_vec=[0 1 2 -1]  value=1  inPortNames=['v'; 'c'; '0'; '1'; '2'; '3'; '4'; '5'; '6'; '7'; '8'; '9'; 'A'; 'B'; 'D'; 'E'; 'F'; 'G'; 'H'; 'I'; 'J'; 'K'; 'L'; 'M'; 'N'; 'O'; 'P'; 'Q'; 'R'; 'S'; 'T'; 'U'; 'W'; 'X'; 'Y'; 'Z']  outPortNames=['v'; 'c'; '0'; '1'; '2'; '3'; '4'; '5'; '6'; '7'; '8'; '9'; 'A'; 'B'; 'D'; 'E'; 'F'; 'G'; 'H'; 'I'; 'J'; 'K'; 'L'; 'M'; 'N'; 'O'; 'P'; 'Q'; 'R'; 'S'; 'T'; 'U'; 'W'; 'X'; 'Y'; 'Z']  dspbaimage=dspba_prim_channel_tall.svg  text=fprintf('In');  style=Optimised  dataSignals=1  foldingEnabled=off  channels=1  sampleRate=200  packetBeginPresent=off  packetBeginEnabled=off  visibilities=dspba_ChannelInVis(gcb)  scheduleOrigin=on  version=20211214
  ChannelIn1 : DSPBAPrim/ChannelIn  primtype=channelin  nInputs=dspba_internal_get_channel_ports(gcb)  nOutputs=dspba_internal_get_channel_ports(gcb)  omode=Inherit via internal rule  otype=sfix(16)  scale=2^-15  rndmethod=Unbiased  factor=1  satmethod=Symmetric  shift_vec=[0 1 2 -1]  value=1  inPortNames=['v'; 'c'; '0'; '1'; '2'; '3'; '4'; '5'; '6'; '7'; '8'; '9'; 'A'; 'B'; 'D'; 'E'; 'F'; 'G'; 'H'; 'I'; 'J'; 'K'; 'L'; 'M'; 'N'; 'O'; 'P'; 'Q'; 'R'; 'S'; 'T'; 'U'; 'W'; 'X'; 'Y'; 'Z']  outPortNames=['v'; 'c'; '0'; '1'; '2'; '3'; '4'; '5'; '6'; '7'; '8'; '9'; 'A'; 'B'; 'D'; 'E'; 'F'; 'G'; 'H'; 'I'; 'J'; 'K'; 'L'; 'M'; 'N'; 'O'; 'P'; 'Q'; 'R'; 'S'; 'T'; 'U'; 'W'; 'X'; 'Y'; 'Z']  dspbaimage=dspba_prim_channel_tall.svg  text=fprintf('In');  style=Optimised  dataSignals=1  foldingEnabled=off  channels=1  sampleRate=200  packetBeginPresent=off  packetBeginEnabled=off  visibilities=dspba_ChannelInVis(gcb)  scheduleOrigin=on  version=20211214
  ChannelOut : DSPBAPrim/ChannelOut  primtype=channelout  nInputs=dspba_internal_get_channel_ports(gcb)  nOutputs=dspba_internal_get_channel_ports(gcb)  omode=Inherit via internal rule  otype=sfix(16)  scale=2^-15  rndmethod=Unbiased  factor=1  satmethod=Symmetric  shift_vec=[0 1 2 -1]  value=1  inPortNames=['v'; 'c'; '0'; '1'; '2'; '3'; '4'; '5'; '6'; '7'; '8'; '9'; 'A'; 'B'; 'D'; 'E'; 'F'; 'G'; 'H'; 'I'; 'J'; 'K'; 'L'; 'M'; 'N'; 'O'; 'P'; 'Q'; 'R'; 'S'; 'T'; 'U'; 'W'; 'X'; 'Y'; 'Z']  outPortNames=['v'; 'c'; '0'; '1'; '2'; '3'; '4'; '5'; '6'; '7'; '8'; '9'; 'A'; 'B'; 'D'; 'E'; 'F'; 'G'; 'H'; 'I'; 'J'; 'K'; 'L'; 'M'; 'N'; 'O'; 'P'; 'Q'; 'R'; 'S'; 'T'; 'U'; 'W'; 'X'; 'Y'; 'Z']  dspbaimage=dspba_prim_channel_tall.svg  text=fprintf('Out%s', AdvDSPBChannelOutDisplay(latency));  style=Optimised  dataSignals=1  foldingEnabled=off  channels=1  sampleRate=200  packetBeginPresent=off  packetBeginEnabled=off  visibilities=dspba_ChannelOutVis(gcb)  latency=3  version=20211214
  ChannelOut1 : DSPBAPrim/ChannelOut  primtype=channelout  nInputs=dspba_internal_get_channel_ports(gcb)  nOutputs=dspba_internal_get_channel_ports(gcb)  omode=Inherit via internal rule  otype=sfix(16)  scale=2^-15  rndmethod=Unbiased  factor=1  satmethod=Symmetric  shift_vec=[0 1 2 -1]  value=1  inPortNames=['v'; 'c'; '0'; '1'; '2'; '3'; '4'; '5'; '6'; '7'; '8'; '9'; 'A'; 'B'; 'D'; 'E'; 'F'; 'G'; 'H'; 'I'; 'J'; 'K'; 'L'; 'M'; 'N'; 'O'; 'P'; 'Q'; 'R'; 'S'; 'T'; 'U'; 'W'; 'X'; 'Y'; 'Z']  outPortNames=['v'; 'c'; '0'; '1'; '2'; '3'; '4'; '5'; '6'; '7'; '8'; '9'; 'A'; 'B'; 'D'; 'E'; 'F'; 'G'; 'H'; 'I'; 'J'; 'K'; 'L'; 'M'; 'N'; 'O'; 'P'; 'Q'; 'R'; 'S'; 'T'; 'U'; 'W'; 'X'; 'Y'; 'Z']  dspbaimage=dspba_prim_channel_tall.svg  text=fprintf('Out%s', AdvDSPBChannelOutDisplay(latency));  style=Optimised  dataSignals=1  foldingEnabled=off  channels=1  sampleRate=200  packetBeginPresent=off  packetBeginEnabled=off  visibilities=dspba_ChannelOutVis(gcb)  latency=6  version=20211214
  Counter : DSPBAPrim/Counter  primtype=counter  nInputs=1  nOutputs=1  omode=Inherit via internal rule  otype=ufix(16)  scale=2^-0  rndmethod=Unbiased  factor=1  satmethod=Symmetric  shift_vec=[0 1 2 -1]  value=[255 256 1]  inPortNames=[' '; ' ';]  outPortNames=[' ']  dspbaimage=dspba_prim.svg  text=fprintf('counter\n[%d %d %d]', value(1), value(2), value(3));  style=Optimised  visibilities=8 + 1024  version=20211007
  Counter1 : DSPBAPrim/Counter  primtype=counter  nInputs=1  nOutputs=1  omode=Inherit via internal rule  otype=ufix(16)  scale=2^-0  rndmethod=Unbiased  factor=1  satmethod=Symmetric  shift_vec=[0 1 2 -1]  value=[255 256 1]  inPortNames=[' '; ' ';]  outPortNames=[' ']  dspbaimage=dspba_prim.svg  text=fprintf('counter\n[%d %d %d]', value(1), value(2), value(3));  style=Optimised  visibilities=8 + 1024  version=20211007
  RegField1 : DSPBAModelBus/RegField  reg_name=DDC_Delay_Comp_offset_ant3_1  reg_rwmode=Read/Write  reg_msb=7  reg_lsb=0  reg_mode=Specify via dialog  reg_type=ufix(8)  reg_scale=2^0  reg_init=DDC_Delay_Comp_Ant3_CC1  reg_desc=Delay Compensation Value  reg_modal=off  reg_desc0=0  reg_desc1=0  reg_desc2=0  reg_desc3=0  reg_desc4=0  reg_desc5=0  reg_desc6=0  reg_desc7=0  reg_addr=7  SampleTime=-1  version=20090407
  RegField2 : DSPBAModelBus/RegField  reg_name=DDC_Delay_Comp_offset_ant4_1  reg_rwmode=Read/Write  reg_msb=7  reg_lsb=0  reg_mode=Specify via dialog  reg_type=ufix(8)  reg_scale=2^0  reg_init=DDC_Delay_Comp_Ant4_CC1  reg_desc=Delay Compensation Value  reg_modal=off  reg_desc0=0  reg_desc1=0  reg_desc2=0  reg_desc3=0  reg_desc4=0  reg_desc5=0  reg_desc6=0  reg_desc7=0  reg_addr=8  SampleTime=-1  version=20090407
  RegField3 : DSPBAModelBus/RegField  reg_name=DDC_Delay_Comp_offset_ant3_2  reg_rwmode=Read/Write  reg_msb=7  reg_lsb=0  reg_mode=Specify via dialog  reg_type=ufix(8)  reg_scale=2^0  reg_init=DDC_Delay_Comp_Ant3_CC2  reg_desc=Delay Compensation Value  reg_modal=off  reg_desc0=0  reg_desc1=0  reg_desc2=0  reg_desc3=0  reg_desc4=0  reg_desc5=0  reg_desc6=0  reg_desc7=0  reg_addr=11  SampleTime=-1  version=20090407
  RegField4 : DSPBAModelBus/RegField  reg_name=DDC_Delay_Comp_offset_ant1_1  reg_rwmode=Read/Write  reg_msb=7  reg_lsb=0  reg_mode=Specify via dialog  reg_type=ufix(8)  reg_scale=2^0  reg_init=DDC_Delay_Comp_Ant1_CC1  reg_desc=Delay Compensation Value  reg_modal=off  reg_desc0=0  reg_desc1=0  reg_desc2=0  reg_desc3=0  reg_desc4=0  reg_desc5=0  reg_desc6=0  reg_desc7=0  reg_addr=5  SampleTime=-1  version=20090407
  RegField6 : DSPBAModelBus/RegField  reg_name=DDC_Delay_Comp_offset_ant2_1  reg_rwmode=Read/Write  reg_msb=7  reg_lsb=0  reg_mode=Specify via dialog  reg_type=ufix(8)  reg_scale=2^0  reg_init=DDC_Delay_Comp_Ant2_CC1  reg_desc=Delay Compensation Value  reg_modal=off  reg_desc0=0  reg_desc1=0  reg_desc2=0  reg_desc3=0  reg_desc4=0  reg_desc5=0  reg_desc6=0  reg_desc7=0  reg_addr=6  SampleTime=-1  version=20090407
  RegField7 : DSPBAModelBus/RegField  reg_name=DDC_Delay_Comp_offset_ant4_2  reg_rwmode=Read/Write  reg_msb=7  reg_lsb=0  reg_mode=Specify via dialog  reg_type=ufix(8)  reg_scale=2^0  reg_init=DDC_Delay_Comp_Ant4_CC2  reg_desc=Delay Compensation Value  reg_modal=off  reg_desc0=0  reg_desc1=0  reg_desc2=0  reg_desc3=0  reg_desc4=0  reg_desc5=0  reg_desc6=0  reg_desc7=0  reg_addr=12  SampleTime=-1  version=20090407
  RegField8 : DSPBAModelBus/RegField  reg_name=DDC_Delay_Comp_offset_ant1_2  reg_rwmode=Read/Write  reg_msb=7  reg_lsb=0  reg_mode=Specify via dialog  reg_type=ufix(8)  reg_scale=2^0  reg_init=DDC_Delay_Comp_Ant1_CC2  reg_desc=Delay Compensation Value  reg_modal=off  reg_desc0=0  reg_desc1=0  reg_desc2=0  reg_desc3=0  reg_desc4=0  reg_desc5=0  reg_desc6=0  reg_desc7=0  reg_addr=9  SampleTime=-1  version=20090407
  RegField9 : DSPBAModelBus/RegField  reg_name=DDC_Delay_Comp_offset_ant2_2  reg_rwmode=Read/Write  reg_msb=7  reg_lsb=0  reg_mode=Specify via dialog  reg_type=ufix(8)  reg_scale=2^0  reg_init=DDC_Delay_Comp_Ant2_CC2  reg_desc=Delay Compensation Value  reg_modal=off  reg_desc0=0  reg_desc1=0  reg_desc2=0  reg_desc3=0  reg_desc4=0  reg_desc5=0  reg_desc6=0  reg_desc7=0  reg_addr=10  SampleTime=-1  version=20090407
  SampleDelay{1..10} (10 alike) : DSPBAPrim/SampleDelay  primtype=sampdelay  nInputs=1  nOutputs=1  omode=Inherit via internal rule  otype=sfix(16)  scale=2^-15  rndmethod=Unbiased  factor=1  satmethod=Symmetric  shift_vec=[0 1 2 -1]  floatPrecision=float32_m23  value=2  inPortNames=[' '; ' ';]  outPortNames=[' ']  dspbaimage=dspba_prim.svg  text=dpoly(1, eye(1,value+1), 'z')  style=Optimised  visibilities=8 + 1024 + 2^17 + 2^18  flexible=off  slackgroup=0  augmented=0  version=20211007  advOptions=[]
  Scope : Scope  NumInputPorts=6
  Scope1 : Scope  NumInputPorts=4
  Sub{,1..7} (8 alike) : DSPBAPrim/Sub  primtype=sub  nInputs=2  nOutputs=1  omode=Specify via dialog  otype=uint(8)  scale=2^0  rndmethod=Unbiased  factor=1  satmethod=Symmetric  shift_vec=[0 1 2 -1]  value=0  inPortNames=['+'; '-';]  outPortNames=[' ']  dspbaimage=dspba_prim.svg  text=fprintf('-');  style=Optimised  visibilities=8+2^17+2^18  floatRounding=correct  advOptions=[]  version=20211007
  Subsystem : Subsystem
  Subsystem1 : Subsystem
  SynthesisInfo : DSPBAPrim/SynthesisInfo  primtype=synthinfo  nInputs=0  nOutputs=0  omode=Inherit via internal rule  otype=sfix(16)  scale=2^-15  rndmethod=Truncate  factor=1  satmethod=Symmetric  shift_vec=[0 1 2 -1]  value=99  inPortNames=[' '; ' ';]  outPortNames=[' ']  dspbaimage=dspba_prim_ctrl.jpg  text=fprintf('Style=%s', style);  style=Scheduled  visibilities=2^15+2^17+2^18+2^19  constraintPair=None  constraintRelation=>  constraintLimit=Latency  modelRefSign=+  modelRef=''  showSchedule=off  simulationMode=Use Global Value  resetMinimization=Conditional - On for ChannelIn/Out only  version=20220106
  TraceAntennaData1 : Subsystem  Commented=on  TreatAsAtomicUnit=on
  TraceAntennaData4 : Subsystem  Commented=on  TreatAsAtomicUnit=on
  altq : Outport
  altv : Outport  Port=2
  altc : Outport  Port=3
  altq1 : Outport  Port=4
  altqv1 : Outport  Port=5
  altc1 : Outport  Port=6
  wires:
  ChannelIn/2 -> Scope1/2, ChannelOut/2
  Counter/1 -> Subsystem/3(WR-add), Sub2/1, Sub1/1, Sub/1, Sub3/1
  RegField4/1 -> Sub/2
  ChannelIn1/1 -> Counter1/1, Subsystem1/1(WR_EN), SampleDelay10/1
  din_a2/1 -> ChannelIn1/3
  vin_a2/1 -> ChannelIn1/1
  ChannelIn1/2 -> ChannelOut1/2
  cin_a2/1 -> ChannelIn1/2
  ChannelOut/3 -> altq/1, Scope/3
  ChannelOut/2 -> altc/1, Scope/2
  ChannelOut/1 -> altv/1, Scope/1
  din_a1/1 -> ChannelIn/3
  vin_a1/1 -> ChannelIn/1
  cin_a1/1 -> ChannelIn/2
  RegField6/1 -> Sub1/2
  RegField1/1 -> Sub2/2
  RegField2/1 -> Sub3/2
  Subsystem/1(Out3) -> ChannelOut/3
  Sub/1 -> SampleDelay4/1
  Sub1/1 -> SampleDelay5/1
  Sub2/1 -> SampleDelay6/1
  Sub3/1 -> SampleDelay7/1
  ChannelIn/3 -> Scope1/3, Subsystem/2(data_in)
  ChannelOut1/3 -> Scope/6, altq1/1
  Subsystem1/1(Out3) -> ChannelOut1/3
  ChannelIn1/3 -> Scope1/4, Subsystem1/2(data_in)
  RegField8/1 -> Sub4/2
  RegField9/1 -> Sub5/2
  RegField3/1 -> Sub6/2
  RegField7/1 -> Sub7/2
  Sub4/1 -> SampleDelay1/1
  Sub5/1 -> SampleDelay2/1
  Sub6/1 -> SampleDelay3/1
  Sub7/1 -> SampleDelay8/1
  ChannelOut1/2 -> Scope/5, altc1/1
  ChannelOut1/1 -> Scope/4, altqv1/1
  SampleDelay4/1 -> Subsystem/4(RD-add1)
  SampleDelay6/1 -> Subsystem/6(RD-add3)
  SampleDelay5/1 -> Subsystem/5(RD-add2)
  SampleDelay7/1 -> Subsystem/7(RD-add4)
  SampleDelay1/1 -> Subsystem1/4(RD-add1)
  SampleDelay2/1 -> Subsystem1/5(RD-add2)
  SampleDelay3/1 -> Subsystem1/6(RD-add3)
  SampleDelay8/1 -> Subsystem1/7(RD-add4)
  Counter1/1 -> Sub7/1, Sub6/1, Sub5/1, Sub4/1, Subsystem1/3(WR-add)
  ChannelIn/1 -> Scope1/1, SampleDelay9/1, Subsystem/1(WR_EN), Counter/1
  SampleDelay10/1 -> ChannelOut1/1
  SampleDelay9/1 -> ChannelOut/1

== system dec_dly_comp/DUT/DUT/Antenna_Gain Delay Compensation/Ant Gain/TraceAntennaData1 ==
  DataIn : Inport
  ChIn : Inport  Port=2
  Enable : EnablePort
  DucAntDataOut : ToWorkspace  VariableName=AntGain_dOut  SampleTime=-1
  DucAntDataOut1 : ToWorkspace  VariableName=AntGain_cOut  SampleTime=-1
  wires:
  DataIn/1 -> DucAntDataOut/1
  ChIn/1 -> DucAntDataOut1/1

== system dec_dly_comp/DUT/DUT/Antenna_Gain Delay Compensation/Ant Gain/TraceAntennaData4 ==
  DataIn : Inport
  ChIn : Inport  Port=2
  Enable : EnablePort
  DucAntDataOut : ToWorkspace  VariableName=AntGain_dIn  SampleTime=-1
  DucAntDataOut1 : ToWorkspace  VariableName=AntGain_cIn  SampleTime=-1
  wires:
  ChIn/1 -> DucAntDataOut1/1
  DataIn/1 -> DucAntDataOut/1

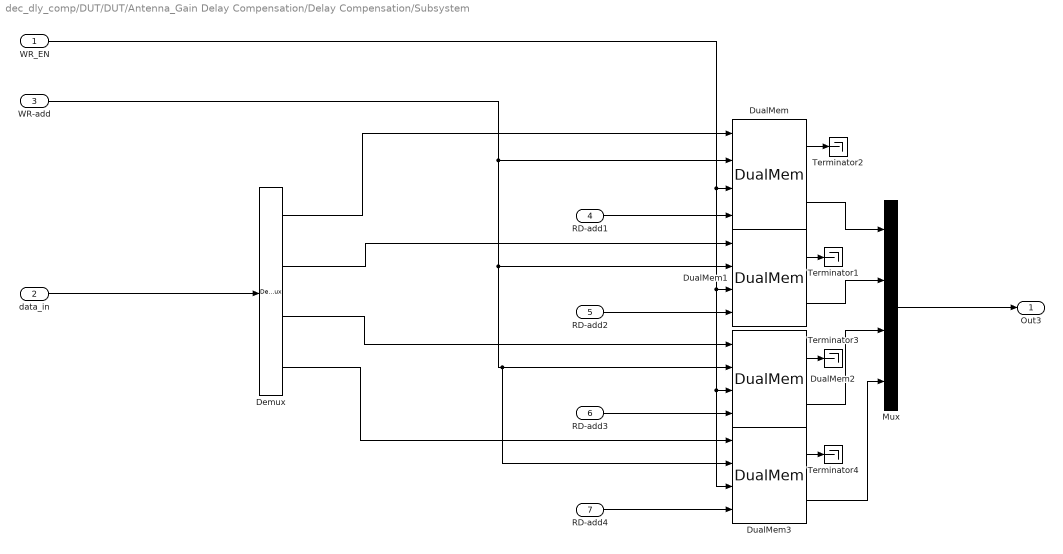
== system dec_dly_comp/DUT/DUT/Antenna_Gain Delay Compensation/Delay Compensation/Subsystem ==
  WR_EN : Inport
  data_in : Inport  Port=2
  WR-add : Inport  Port=3
  RD-add1 : Inport  Port=4
  RD-add2 : Inport  Port=5
  RD-add3 : Inport  Port=6
  RD-add4 : Inport  Port=7
  Demux : Demux
  DualMem{,1..3} (4 alike) : DSPBAPrim/DualMem  primtype=dualmem  nInputs=4  nOutputs=2  omode=Inherit via internal rule  otype=sfix(16)  scale=2^-15  rndmethod=Unbiased  factor=1  satmethod=Symmetric  shift_vec=[0 1 2 -1]  value=[zeros(256, 1)]  inPortNames=['d1'; 'a1'; 'w1'; 'd2'; 'a2'; 'w2']  outPortNames=['q1'; 'q2']  dspbaimage=dspba_prim_tall.svg  text=fprintf('dmem%s',AdvDSPBDMemDisplay(UseDontCare));  style=Optimised  visibilities=8 + 1024 + 2^17 + 2^18  UseDontCare=on  TwinWritePorts=off  init=on  ProvideReadAccess=off  version=20211007
  Mux : Mux
  Terminator{1..4} (4 alike) : Terminator
  Out3 : Outport
  wires:
  WR-add/1 -> DualMem/2, DualMem1/2, DualMem2/2, DualMem3/2
  DualMem1/2 -> Mux/2
  WR_EN/1 -> DualMem2/3, DualMem3/3, DualMem1/3, DualMem/3
  DualMem3/1 -> Terminator4/1
  RD-add2/1 -> DualMem1/4
  DualMem2/2 -> Mux/3
  Demux/4 -> DualMem3/1
  DualMem/1 -> Terminator2/1
  Demux/3 -> DualMem2/1
  RD-add3/1 -> DualMem2/4
  DualMem/2 -> Mux/1
  DualMem3/2 -> Mux/4
  Demux/2 -> DualMem1/1
  Demux/1 -> DualMem/1
  RD-add4/1 -> DualMem3/4
  Mux/1 -> Out3/1
  RD-add1/1 -> DualMem/4
  data_in/1 -> Demux/1
  DualMem2/1 -> Terminator3/1
  DualMem1/1 -> Terminator1/1

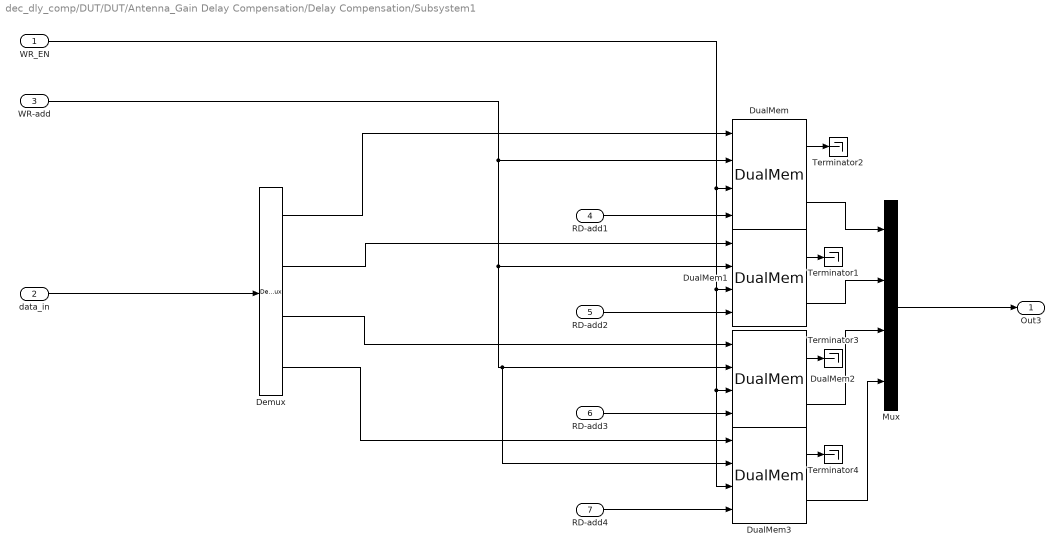
== system dec_dly_comp/DUT/DUT/Antenna_Gain Delay Compensation/Delay Compensation/Subsystem1 ==
  WR_EN : Inport
  data_in : Inport  Port=2
  WR-add : Inport  Port=3
  RD-add1 : Inport  Port=4
  RD-add2 : Inport  Port=5
  RD-add3 : Inport  Port=6
  RD-add4 : Inport  Port=7
  Demux : Demux
  DualMem{,1..3} (4 alike) : DSPBAPrim/DualMem  primtype=dualmem  nInputs=4  nOutputs=2  omode=Inherit via internal rule  otype=sfix(16)  scale=2^-15  rndmethod=Unbiased  factor=1  satmethod=Symmetric  shift_vec=[0 1 2 -1]  value=[zeros(256, 1)]  inPortNames=['d1'; 'a1'; 'w1'; 'd2'; 'a2'; 'w2']  outPortNames=['q1'; 'q2']  dspbaimage=dspba_prim_tall.svg  text=fprintf('dmem%s',AdvDSPBDMemDisplay(UseDontCare));  style=Optimised  visibilities=8 + 1024 + 2^17 + 2^18  UseDontCare=on  TwinWritePorts=off  init=on  ProvideReadAccess=off  version=20211007
  Mux : Mux
  Terminator{1..4} (4 alike) : Terminator
  Out3 : Outport
  wires:
  DualMem1/1 -> Terminator1/1
  DualMem2/1 -> Terminator3/1
  data_in/1 -> Demux/1
  RD-add1/1 -> DualMem/4
  Mux/1 -> Out3/1
  RD-add4/1 -> DualMem3/4
  Demux/1 -> DualMem/1
  Demux/2 -> DualMem1/1
  DualMem3/2 -> Mux/4
  DualMem/2 -> Mux/1
  RD-add3/1 -> DualMem2/4
  Demux/3 -> DualMem2/1
  DualMem/1 -> Terminator2/1
  Demux/4 -> DualMem3/1
  DualMem2/2 -> Mux/3
  RD-add2/1 -> DualMem1/4
  DualMem3/1 -> Terminator4/1
  WR_EN/1 -> DualMem/3, DualMem1/3, DualMem3/3, DualMem2/3
  DualMem1/2 -> Mux/2
  WR-add/1 -> DualMem3/2, DualMem2/2, DualMem1/2, DualMem/2
